simulink model "MMC_Control_PLECS_V2_R2016a"  (R2016a)
settings: Solver=VariableStepAuto  SolverMode=SingleTasking  StartTime=0.0  StopTime=0.02  FixedStep=sim_Ts  RelTol=1e-3
undefined symbols (not defined in the file): plecs
settings Model: Creator=jason  LastModifiedBy=Francis Chen
settings DebuggingCC: SFUnexpectedBacktrackingDiag=error  SFNoUnconditionalDefaultTransitionDiag=error
settings SFSimCC: SimUseLocalCustomCode=on
settings RTWCC: RTWUseLocalCustomCode=on
settings GRTTargetCC: TargetLangStandard=C99 (ISO)  GeneratePreprocessorConditionals=Use local settings
settings ConfigComp: CovMetricSettings=dwe  CovHtmlReporting=off  CovSaveCumulativeToWorkspaceVar=off  CovSaveSingleToWorkspaceVar=off  CovExternalEMLEnable=on

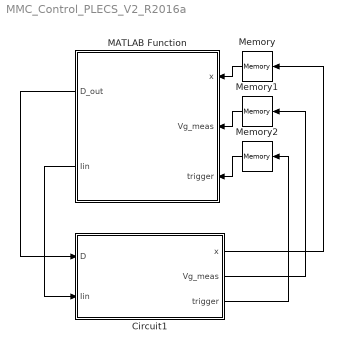
== system MMC_Control_PLECS_V2_R2016a ==
  Circuit1 : Subsystem  LoadFcn=plecs('sl', 200);  InitFcn=plecs('sl', 214);  StartFcn=plecs('sl', 208);  StopFcn=plecs('sl', 209);  mask(PlecsCircuit){PLECSData=<binary blob, 36264 chars, not shown>}
      mask prompts: PLECSData "PLECS Data (Do not delete or modify!)"
      mask init:
      | % PLACE CUSTOM INITIALIZATIONS ABOVE
      | % DO NOT REMOVE
      | plecs('sl', 215);
      | % DO NOT REMOVE
      settings: CopyFcn=plecs('sl', 203);  DeleteFcn=plecs('sl', 205);  UndoDeleteFcn=plecs('sl', 206);  PreSaveFcn=plecs('sl', 211);  PostSaveFcn=plecs('sl', 201);  NameChangeFcn=plecs('sl', 210);  DestroyFcn=plecs('sl', 207);  PreCopyFcn=plecs('sl', 216);  OpenFcn=plecs('sl', 202);  ErrorFcn=plerrorfcn
      mask Help: web(['file:///' fullfile(plecsdoc, 'creatingacircuit.html')])
      mask Display: disp('PLECS\nCircuit')
  MATLAB Function : MATLAB Function  TreatAsAtomicUnit=on
  Memory : Memory  X0=[50,50,50,4,4,4];  InheritSampleTime=on
  Memory1 : Memory  X0=[0,0,0];  InheritSampleTime=on
  Memory2 : Memory  InheritSampleTime=on
  wires:
  Circuit1/3(trigger) -> Memory2/1
  Circuit1/2(Vg_meas) -> Memory1/1
  Circuit1/1(x) -> Memory/1
  MATLAB Function/2(Iin) -> Circuit1/2(Iin)
  MATLAB Function/1(D_out) -> Circuit1/1(D)
  Memory/1 -> MATLAB Function/1(x)
  Memory1/1 -> MATLAB Function/2(Vg_meas)
  Memory2/1 -> MATLAB Function/3(trigger)

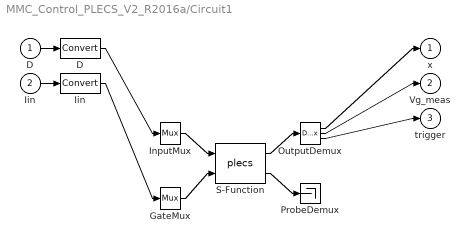
== system MMC_Control_PLECS_V2_R2016a/Circuit1 ==
  D : Inport  PortDimensions=6
  Iin : Inport  Port=2  PortDimensions=3
  " D " : DataTypeConversion  SaturateOnIntegerOverflow=on  RndMeth=Zero
  " GateMux " : Mux  Inputs=[ 3 ]
  " Iin " : DataTypeConversion  SaturateOnIntegerOverflow=on  RndMeth=Zero
  " InputMux " : Mux  Inputs=[ 6 ]
  " OutputDemux " : Demux  Outputs=[ 6 3 1 ]
  " ProbeDemux " : Terminator
  " S-Function " : S-Function  FunctionName=plecs  SFunctionDeploymentMode=off  EnableBusSupport=off
  x : Outport  PortDimensions=6
  Vg_meas : Outport  Port=2  PortDimensions=3
  trigger : Outport  Port=3  PortDimensions=1
  wires:
  " InputMux "/1 -> " S-Function "/1
  " GateMux "/1 -> " S-Function "/2
  " S-Function "/1 -> " OutputDemux "/1
  " S-Function "/2 -> " ProbeDemux "/1
  D/1 -> " D "/1
  " D "/1 -> " InputMux "/1
  Iin/1 -> " Iin "/1
  " Iin "/1 -> " GateMux "/1
  " OutputDemux "/1 -> x/1
  " OutputDemux "/2 -> Vg_meas/1
  " OutputDemux "/3 -> trigger/1

== matlab function MMC_Control_PLECS_V2_R2016a/MATLAB Function ==
  data: x input; D_out output; Iin output; Vg_meas input; trigger input; nom parameter
function [D_out, Iin] = MMC_control(x, Vg_meas, trigger,nom)



persistent D_out_val err_int_val 
if isempty(D_out_val)
    D_out_val = [0.5; 0.5; 0.5; 0.5; 0.5; 0.5];
    err_int_val = zeros(5,1);
end

% Some nominal values 
Vpv  = 50; 
Ipv = 3;
Iin = [Ipv; Ipv; Ipv];

if trigger    
Vg_peak = 40; 
Nstate = 6; 
Nout = 5; 

phi     = asin(Vg_meas(1)/Vg_peak);
tstep      = ceil(interp1(nom.phi,nom.id,phi));
% xnom    = nom.x(tstep,:)'; 
xnom    =  [Vpv,Vpv,Vpv,4,4,4]';
% K  = nom.K   (tstep,:,:); 
% K  = reshape (K,Nstate,Nstate+Nout);

Ki =[286.941473237871,-54.8067087595862,58.5030731672240,-190.788522691937,473.296966681327;80.9087565771101,-50.3855670178550,293.826775986482,-402.976033800235,-267.191588405387;286.941473237871,58.5030731672242,-54.8067087595864,473.296966681323,-190.788522691940;80.9087565771100,293.826775986482,-50.3855670178552,-267.191588405391,-402.976033800237;-58.6257816982106,292.482316754915,61.5797556773875,-35.2328058235777,493.068238154840;-58.6257816982106,61.5797556773877,292.482316754914,493.068238154838,-35.2328058235770];
Kp = [-0.0228163508348687,0.00140297609429514,0.00111096015507632,0.0560401150484045,-0.000444350700924729,-0.00128826948572575;0.00235478276817947,0.00648043131429393,-0.0186767823351992,0.0570351731388870,0.000317094638182779,0.00379953433664691;-0.0228163508348686,0.00111096015507634,0.00140297609429515,-0.000444350700924680,0.0560401150484045,-0.00128826948572576;0.00235478276817955,-0.0186767823351992,0.00648043131429395,0.000317094638182799,0.0570351731388871,0.00379953433664692;0.00202848104708184,-0.0241190162211596,0.000746181489114811,-0.000787865523496387,-0.000554252772121364,0.0537247696573178;0.00202848104708183,0.000746181489114776,-0.0241190162211595,-0.000554252772121348,-0.000787865523496417,0.0537247696573178];

 

% Ki = K       (:,1:Nout); 
% Kp = K       (:,Nout+1:end);

Igd = Vg_meas ./ 5.3333;
% yd  = abs(xnom(1:end-1)); % last point is not tracked (5 measurements to track)
yd = [50; 50 ;50; abs(Igd(1:2))];

tcy = 1/nom.fsw;
% D0            = nom.D (tstep,:)'; %Nominal Duty Cycle
D0            = 0.5*ones(Nstate,1); 
y             = abs(x(1:5));
state   =   abs(x) - xnom; 
err     =   yd - y; % only care about absolute value 
err_int =   err*tcy  + err_int_val;

dD      = - Kp*state - Ki*err_int;
D       =   D0+dD;  % pay close attention to the sign!
D       =   max(min(D,0.999),0.001);

Veps = 0;%1.1233e-6;
D(1:2) = sign(Vg_meas(1)+Veps)*D(1:2); 
D(3:4) = sign(Vg_meas(2)+Veps)*D(3:4); 
D(5:6) = sign(Vg_meas(3)+Veps)*D(5:6); 


    D_out = D;
    D_out_val = D;
    err_int_val = err_int;
else
    D_out = D_out_val;
end


end %function
